simulink model "TiltRotorQuad"  (R2022b)
settings: Solver=VariableStepAuto  StartTime=0.0  StopTime=10  RelTol=1e-3
values from neighbouring files (symbols this model uses):
  k = 7.075135827e-05    [QuadSimParameters.mat]
undefined symbols (not defined in the file or in its folder): X, Y, Z
libraries: sm_lib x46, nesl_utility x25
(part 3 of 3)

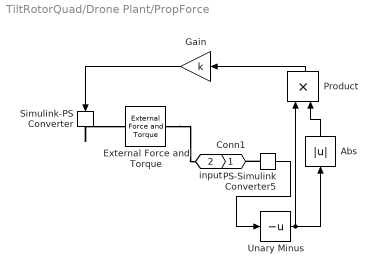
== system TiltRotorQuad/Drone Plant/PropForce ==
  Abs : Abs  SaturateOnIntegerOverflow=off
  External Force and Torque : sm_lib/Forces and Torques/External Force and Torque  ForceResolutionFrame=AttachedFrame  EnableForceX=off  EnableForceY=off  EnableForceZ=on  EnableForce=off  TorqueResolutionFrame=AttachedFrame  EnableTorqueX=off  EnableTorqueY=off  EnableTorqueZ=off  EnableTorque=off
  Gain : Gain  Gain=k
  PS-Simulink Converter5 : nesl_utility/PS-Simulink Converter  PhysicalDomain=network_engine_domain  SubClassName=ps_output  LeftPortType=input  RightPortType=output  PseudoPeriodic=off  Frequencies=[]  VectorFormat=inherit  Unit=inherit  AffineConversion=off
  Product : Product
  Simulink-PS Converter : nesl_utility/Simulink-PS Converter  PhysicalDomain=network_engine_domain  SubClassName=ps_input  LeftPortType=input  RightPortType=output  PseudoPeriodic=off  Frequencies=[]  NoiseDistribution=none  NoiseParameters=[]  Unit=1  AffineConversion=off  FilteringAndDerivatives=provide  SimscapeFilterOrder=1  InputFilterTimeConstant=0.001  UdotUserProvided=0
  Unary Minus : UnaryMinus
  Conn1 : PMIOPort  Side=Right
  input : PMIOPort  Port=2  Side=Left
  wires:
  Gain/1 -> Simulink-PS Converter/1
  Abs/1 -> Product/2
  Product/1 -> Gain/1
  Unary Minus/1 -> Product/1, Abs/1
  PS-Simulink Converter5/1 -> Unary Minus/1
  connections:
  External Force and Torque/RConn1 -- Conn1/RConn1
  Simulink-PS Converter/RConn1 -- External Force and Torque/LConn1
  PS-Simulink Converter5/LConn1 -- input/RConn1

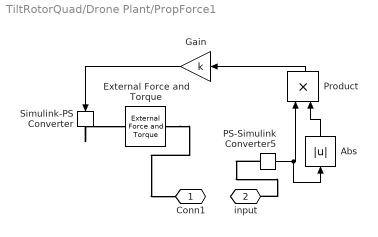
== system TiltRotorQuad/Drone Plant/PropForce1 ==
  Abs : Abs  SaturateOnIntegerOverflow=off
  External Force and Torque : sm_lib/Forces and Torques/External Force and Torque  ForceResolutionFrame=AttachedFrame  EnableForceX=off  EnableForceY=off  EnableForceZ=on  EnableForce=off  TorqueResolutionFrame=AttachedFrame  EnableTorqueX=off  EnableTorqueY=off  EnableTorqueZ=off  EnableTorque=off
  Gain : Gain  Gain=k
  PS-Simulink Converter5 : nesl_utility/PS-Simulink Converter  PhysicalDomain=network_engine_domain  SubClassName=ps_output  LeftPortType=input  RightPortType=output  PseudoPeriodic=off  Frequencies=[]  VectorFormat=inherit  Unit=inherit  AffineConversion=off
  Product : Product
  Simulink-PS Converter : nesl_utility/Simulink-PS Converter  PhysicalDomain=network_engine_domain  SubClassName=ps_input  LeftPortType=input  RightPortType=output  PseudoPeriodic=off  Frequencies=[]  NoiseDistribution=none  NoiseParameters=[]  Unit=1  AffineConversion=off  FilteringAndDerivatives=provide  SimscapeFilterOrder=1  InputFilterTimeConstant=0.001  UdotUserProvided=0
  Conn1 : PMIOPort  Side=Right
  input : PMIOPort  Port=2  Side=Left
  wires:
  Product/1 -> Gain/1
  PS-Simulink Converter5/1 -> Abs/1, Product/1
  Abs/1 -> Product/2
  Gain/1 -> Simulink-PS Converter/1
  connections:
  PS-Simulink Converter5/LConn1 -- input/RConn1
  Simulink-PS Converter/RConn1 -- External Force and Torque/LConn1
  External Force and Torque/RConn1 -- Conn1/RConn1

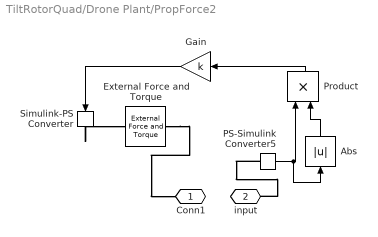
== system TiltRotorQuad/Drone Plant/PropForce2 ==
  Abs : Abs  SaturateOnIntegerOverflow=off
  External Force and Torque : sm_lib/Forces and Torques/External Force and Torque  ForceResolutionFrame=AttachedFrame  EnableForceX=off  EnableForceY=off  EnableForceZ=on  EnableForce=off  TorqueResolutionFrame=AttachedFrame  EnableTorqueX=off  EnableTorqueY=off  EnableTorqueZ=off  EnableTorque=off
  Gain : Gain  Gain=k
  PS-Simulink Converter5 : nesl_utility/PS-Simulink Converter  PhysicalDomain=network_engine_domain  SubClassName=ps_output  LeftPortType=input  RightPortType=output  PseudoPeriodic=off  Frequencies=[]  VectorFormat=inherit  Unit=inherit  AffineConversion=off
  Product : Product
  Simulink-PS Converter : nesl_utility/Simulink-PS Converter  PhysicalDomain=network_engine_domain  SubClassName=ps_input  LeftPortType=input  RightPortType=output  PseudoPeriodic=off  Frequencies=[]  NoiseDistribution=none  NoiseParameters=[]  Unit=1  AffineConversion=off  FilteringAndDerivatives=provide  SimscapeFilterOrder=1  InputFilterTimeConstant=0.001  UdotUserProvided=0
  Conn1 : PMIOPort  Side=Right
  input : PMIOPort  Port=2  Side=Left
  wires:
  Gain/1 -> Simulink-PS Converter/1
  Abs/1 -> Product/2
  PS-Simulink Converter5/1 -> Product/1, Abs/1
  Product/1 -> Gain/1
  connections:
  External Force and Torque/RConn1 -- Conn1/RConn1
  Simulink-PS Converter/RConn1 -- External Force and Torque/LConn1
  PS-Simulink Converter5/LConn1 -- input/RConn1

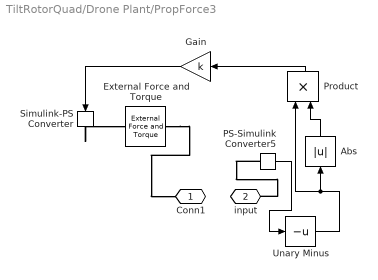
== system TiltRotorQuad/Drone Plant/PropForce3 ==
  Abs : Abs  SaturateOnIntegerOverflow=off
  External Force and Torque : sm_lib/Forces and Torques/External Force and Torque  ForceResolutionFrame=AttachedFrame  EnableForceX=off  EnableForceY=off  EnableForceZ=on  EnableForce=off  TorqueResolutionFrame=AttachedFrame  EnableTorqueX=off  EnableTorqueY=off  EnableTorqueZ=off  EnableTorque=off
  Gain : Gain  Gain=k
  PS-Simulink Converter5 : nesl_utility/PS-Simulink Converter  PhysicalDomain=network_engine_domain  SubClassName=ps_output  LeftPortType=input  RightPortType=output  PseudoPeriodic=off  Frequencies=[]  VectorFormat=inherit  Unit=inherit  AffineConversion=off
  Product : Product
  Simulink-PS Converter : nesl_utility/Simulink-PS Converter  PhysicalDomain=network_engine_domain  SubClassName=ps_input  LeftPortType=input  RightPortType=output  PseudoPeriodic=off  Frequencies=[]  NoiseDistribution=none  NoiseParameters=[]  Unit=1  AffineConversion=off  FilteringAndDerivatives=provide  SimscapeFilterOrder=1  InputFilterTimeConstant=0.001  UdotUserProvided=0
  Unary Minus : UnaryMinus
  Conn1 : PMIOPort  Side=Right
  input : PMIOPort  Port=2  Side=Left
  wires:
  Product/1 -> Gain/1
  Abs/1 -> Product/2
  Gain/1 -> Simulink-PS Converter/1
  PS-Simulink Converter5/1 -> Unary Minus/1
  Unary Minus/1 -> Abs/1, Product/1
  connections:
  PS-Simulink Converter5/LConn1 -- input/RConn1
  Simulink-PS Converter/RConn1 -- External Force and Torque/LConn1
  External Force and Torque/RConn1 -- Conn1/RConn1

== matlab function TiltRotorQuad/Drone Plant/MATLAB Function ==
  data: u input; alpha output
function alpha = fcn(u)

alpha = 180*u(2)/pi;

== matlab function TiltRotorQuad/Drone Plant/MATLAB Function2 ==
  data: u input; gamma output
function gamma = fcn(u)

gamma = 180*u(1)/pi;

== matlab function TiltRotorQuad/Drone Plant/MATLAB Function1 ==
  data: u input; beta output
function beta = fcn(u)

beta = 180*u(2)/pi;
